simulink model "mdl_filter_complementary_16b"  (R2016b)
settings: Solver=FixedStepAuto  StartTime=0.0  StopTime=30  FixedStep=1e-2  RelTol=1e-3
values from neighbouring files (symbols this model uses):
  w0 = 0.6    [mdl_filter_complementary_par.m]
undefined symbols (not defined in the file or in its folder): Ag_phi_rad, Ag_theta_rad, AgVel_p_radPerScnd, AgVel_q_radPerScnd
libraries: simulink x3
settings Model: Creator=Nu  LastModifiedBy=Nu

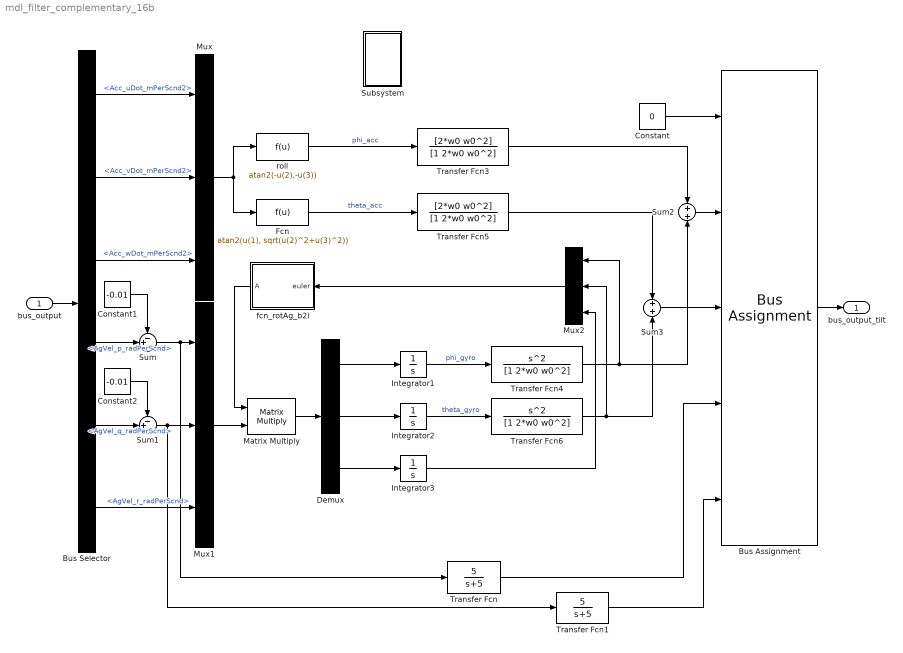
== system mdl_filter_complementary_16b ==
  bus_output : Inport  OutDataTypeStr=Bus: mdl_output
  Bus Assignment : BusAssignment  AssignedSignals=Ag_phi_rad,Ag_theta_rad,AgVel_p_radPerScnd,AgVel_q_radPerScnd
  Bus Selector : BusSelector  OutputSignals=Acc_uDot_mPerScnd2,Acc_vDot_mPerScnd2,Acc_wDot_mPerScnd2,AgVel_p_radPerScnd,AgVel_q_radPerScnd,AgVel_r_radPerScnd
  Constant : Constant  Value=0  OutDataTypeStr=Bus: mdl_statesExt
  Constant1 : Constant  Value=-0.01
  Constant2 : Constant  Value=-0.01
  Demux : Demux  Outputs=3
  Fcn : Fcn  Expr=atan2(u(1), sqrt(u(2)^2+u(3)^2))
  Integrator1 : Integrator
  Integrator2 : Integrator
  Integrator3 : Integrator
  Matrix Multiply : Product  Multiplication=Matrix(*)
  Mux : Mux  Inputs=3
  Mux1 : Mux  Inputs=3
  Mux2 : Mux  Inputs=3
  Subsystem : Subsystem
  Sum : Sum  Inputs=-+|
  Sum1 : Sum  Inputs=-+|
  Sum2 : Sum
  Sum3 : Sum
  Transfer Fcn : TransferFcn  Numerator=[5]  Denominator=[1 5]
  Transfer Fcn1 : TransferFcn  Numerator=[5]  Denominator=[1 5]
  Transfer Fcn3 : TransferFcn  Numerator=[2*w0 w0^2]  Denominator=[1 2*w0 w0^2]
  Transfer Fcn4 : TransferFcn  Numerator=[1 0 0]  Denominator=[1 2*w0 w0^2]
  Transfer Fcn5 : TransferFcn  Numerator=[2*w0 w0^2]  Denominator=[1 2*w0 w0^2]
  Transfer Fcn6 : TransferFcn  Numerator=[1 0 0]  Denominator=[1 2*w0 w0^2]
  fcn_rotAg_b2i : MATLAB Function  TreatAsAtomicUnit=on
  roll : Fcn  Expr=atan2(-u(2),-u(3))
  "bus_output_tilt " : Outport  OutDataTypeStr=Bus: mdl_statesExt
  wires:
  Bus Selector/1 -> Mux/1  "<Acc_uDot_mPerScnd2>"
  Bus Selector/2 -> Mux/2  "<Acc_vDot_mPerScnd2>"
  Bus Selector/3 -> Mux/3  "<Acc_wDot_mPerScnd2>"
  Mux/1 -> roll/1, Fcn/1
  roll/1 -> Transfer Fcn3/1  "phi_acc"
  Integrator1/1 -> Transfer Fcn4/1  "phi_gyro"
  Transfer Fcn3/1 -> Sum2/1
  Transfer Fcn4/1 -> Mux2/1, Sum2/2
  Fcn/1 -> Transfer Fcn5/1  "theta_acc"
  Integrator2/1 -> Transfer Fcn6/1  "theta_gyro"
  Transfer Fcn5/1 -> Sum3/1
  Transfer Fcn6/1 -> Mux2/2, Sum3/2
  Sum3/1 -> Bus Assignment/3
  Bus Selector/6 -> Mux1/3  "<AgVel_r_radPerScnd>"
  bus_output/1 -> Bus Selector/1
  Sum1/1 -> Transfer Fcn1/1, Mux1/2
  Constant/1 -> Bus Assignment/1
  Sum2/1 -> Bus Assignment/2
  Bus Assignment/1 -> "bus_output_tilt "/1
  Sum/1 -> Transfer Fcn/1, Mux1/1
  Mux1/1 -> Matrix Multiply/2
  fcn_rotAg_b2i/1(A) -> Matrix Multiply/1
  Matrix Multiply/1 -> Demux/1
  Demux/1 -> Integrator1/1
  Demux/2 -> Integrator2/1
  Demux/3 -> Integrator3/1
  Integrator3/1 -> Mux2/3
  Mux2/1 -> fcn_rotAg_b2i/1(euler)
  Bus Selector/4 -> Sum/2  "<AgVel_p_radPerScnd>"
  Constant1/1 -> Sum/1
  Bus Selector/5 -> Sum1/2  "<AgVel_q_radPerScnd>"
  Constant2/1 -> Sum1/1
  Transfer Fcn/1 -> Bus Assignment/4
  Transfer Fcn1/1 -> Bus Assignment/5

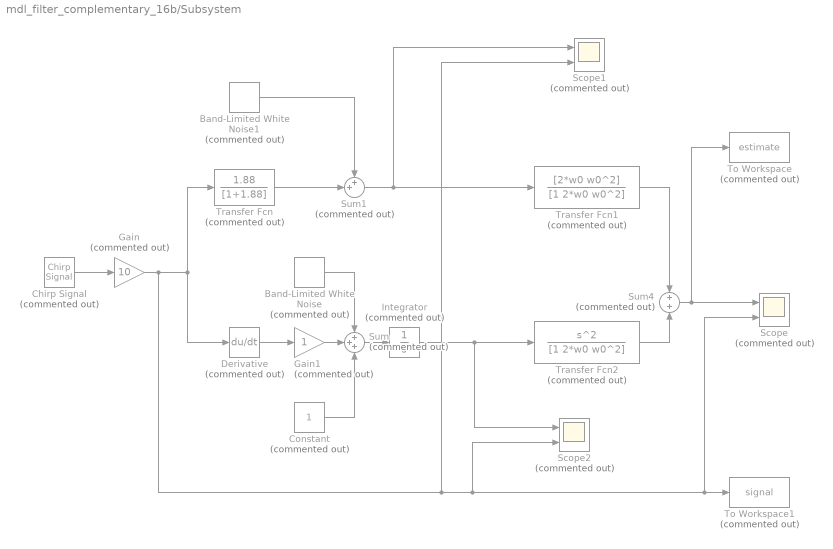
== system mdl_filter_complementary_16b/Subsystem ==
  Band-Limited White Noise : simulink/Sources/Band-Limited White Noise  Commented=on  Cov=[0.1]  Ts=0.1  seed=[23341]
  Band-Limited White Noise1 : simulink/Sources/Band-Limited White Noise  Commented=on  Cov=[0.1]  Ts=0.1  seed=[23341]
  Chirp Signal : simulink/Sources/Chirp Signal  Commented=on  f1=0.1  T=100  f2=0.05
  Constant : Constant  Commented=on
  Derivative : Derivative  Commented=on
  Gain : Gain  Commented=on  Gain=10
  Gain1 : Gain  Commented=on
  Integrator : Integrator  Commented=on
  Scope : Scope  Commented=on  NumInputPorts=2
  Scope1 : Scope  Commented=on  NumInputPorts=2
  Scope2 : Scope  Commented=on  NumInputPorts=2
  Sum : Sum  Commented=on  Inputs=+++
  Sum1 : Sum  Commented=on  Inputs=++|
  Sum4 : Sum  Commented=on
  To Workspace : ToWorkspace  Commented=on  VariableName=estimate  SampleTime=-1
  To Workspace1 : ToWorkspace  Commented=on  VariableName=signal  SampleTime=-1
  Transfer Fcn : TransferFcn  Commented=on  Numerator=[1.88]  Denominator=[1+1.88]
  Transfer Fcn1 : TransferFcn  Commented=on  Numerator=[2*w0 w0^2]  Denominator=[1 2*w0 w0^2]
  Transfer Fcn2 : TransferFcn  Commented=on  Numerator=[1 0 0]  Denominator=[1 2*w0 w0^2]
  wires:
  Chirp Signal/1 -> Gain/1
  Transfer Fcn/1 -> Sum1/2
  Transfer Fcn1/1 -> Sum4/1
  Transfer Fcn2/1 -> Sum4/2
  Band-Limited White Noise/1 -> Sum/1
  Constant/1 -> Sum/3
  Sum4/1 -> To Workspace/1, Scope/1
  Gain/1 -> Scope1/2, Scope2/2, Scope/2, To Workspace1/1, Transfer Fcn/1, Derivative/1
  Sum/1 -> Integrator/1
  Integrator/1 -> Scope2/1, Transfer Fcn2/1
  Sum1/1 -> Scope1/1, Transfer Fcn1/1
  Derivative/1 -> Gain1/1
  Gain1/1 -> Sum/2
  Band-Limited White Noise1/1 -> Sum1/1

== matlab function mdl_filter_complementary_16b/fcn_rotAg_b2i ==
  data: euler input size=3; A output
function A = fcn(euler)

phi     = euler(1);
theta   = euler(2);
psi     = euler(3);

A       = mdl_rotKarman_zyx_b2i(phi, theta, psi);
